simulink model "ClusterMG_1_SG"  (R2020a)
settings: Solver=FixedStepAuto  StartTime=0.0  StopTime=Tss  RelTol=1e-5  AbsTol=1e-5  EnableMultiTasking=on
values from neighbouring files (symbols this model uses):
  KA = K_sweep(cont)    [fault_tesis_1_SG.m]
  Ti = 1.5e-4    (= 0.00015)    [fault_tesis_1_SG.m]
  Tof = 1    [fault_tesis_1_SG.m]
undefined symbols (not defined in the file or in its folder): DiscIntNeverNeededParam, sigbuilder_block
libraries: powerlib x88, powerlib_meascontrol x49, simulink x20, spsExcitationSystemModel x1
(part 3 of 3)

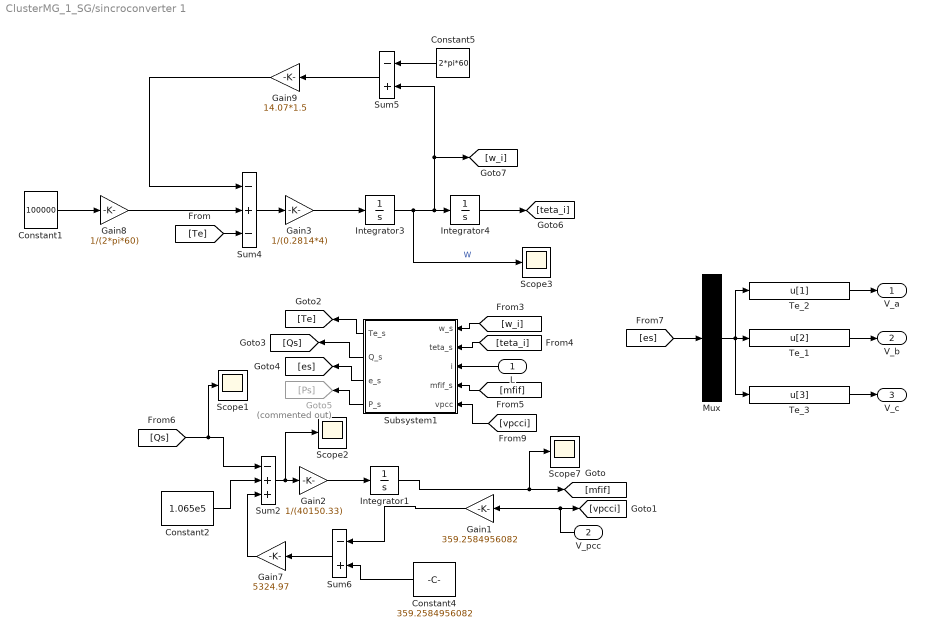
== system ClusterMG_1_SG/sincroconverter 1 ==
  L : Inport
  V_pcc : Inport  Port=2
  Constant1 : Constant  Value=100000
  Constant2 : Constant  Value=1.065e5
  Constant4 : Constant  Value=359.2584956082
  Constant5 : Constant  Value=2*pi*60
  Gain1 : Gain  Gain=359.2584956082
  Gain2 : Gain  Gain=1/(40150.33)
  Gain3 : Gain  Gain=1/(0.2814*4)
  Gain7 : Gain  Gain=5324.97
  Gain8 : Gain  Gain=1/(2*pi*60)
  Gain9 : Gain  Gain=14.07*1.5
  Goto5 : Goto  Commented=on  GotoTag=Ps
  Integrator1 : Integrator
  Integrator3 : Integrator  InitialCondition=376.9911
  Integrator4 : Integrator
  Mux : Mux  Inputs=1
  Scope{1..3,7} (4 alike) : Scope
  Subsystem1 : Subsystem
  Sum2 : Sum  Inputs=-++  InputSameDT=on  SaturateOnIntegerOverflow=on  OutDataTypeStr=Inherit: Same as first input
  Sum4 : Sum  Inputs=-+-  InputSameDT=on  SaturateOnIntegerOverflow=on  OutDataTypeStr=Inherit: Same as first input
  Sum5 : Sum  Inputs=-+  InputSameDT=on  SaturateOnIntegerOverflow=on  OutDataTypeStr=Inherit: Same as first input
  Sum6 : Sum  Inputs=-+  InputSameDT=on  SaturateOnIntegerOverflow=on  OutDataTypeStr=Inherit: Same as first input
  Te_1 : Fcn  Expr=u[2]
  Te_2 : Fcn  Expr=u[1]
  Te_3 : Fcn  Expr=u[3]
  V_a : Outport  VectorParamsAs1DForOutWhenUnconnected=off
  V_b : Outport  Port=2  VectorParamsAs1DForOutWhenUnconnected=off
  V_c : Outport  Port=3  VectorParamsAs1DForOutWhenUnconnected=off
  wires:
  Te_2/1 -> V_a/1
  Mux/1 -> Te_3/1, Te_2/1, Te_1/1
  Te_1/1 -> V_b/1
  Te_3/1 -> V_c/1
  [w_i] -> Subsystem1/1(w_s)
  [teta_i] -> Subsystem1/2(teta_s)
  [mfif] -> Subsystem1/4(mfif_s)
  Subsystem1/1(Te_s) -> [Te]
  Subsystem1/3(e_s) -> [es]
  Gain9/1 -> Sum4/1
  Sum4/1 -> Gain3/1
  Constant5/1 -> Sum5/1
  Integrator4/1 -> [teta_i]
  Sum5/1 -> Gain9/1
  Gain8/1 -> Sum4/2
  Gain3/1 -> Integrator3/1
  [Te] -> Sum4/3
  Gain7/1 -> Sum2/3
  Constant4/1 -> Sum6/2
  Gain2/1 -> Integrator1/1
  Sum6/1 -> Gain7/1
  Sum2/1 -> Scope2/1, Gain2/1
  L/1 -> Subsystem1/3(i)
  [es] -> Mux/1
  [Qs] -> Scope1/1, Sum2/1
  Subsystem1/4(P_s) -> Goto5/1
  Subsystem1/2(Q_s) -> [Qs]
  Constant2/1 -> Sum2/2
  Constant1/1 -> Gain8/1
  Integrator3/1 -> Scope3/1, Sum5/2, [w_i], Integrator4/1  "W"
  V_pcc/1 -> [vpcci], Gain1/1
  Integrator1/1 -> Scope7/1, [mfif]
  [vpcci] -> Subsystem1/5(vpcc)
  Gain1/1 -> Sum6/1

== system ClusterMG_1_SG/PLL/abc - qd ==
  a : Inport
  b : Inport  Port=2
  c : Inport  Port=3
  Gain : Gain  Gain=2/3
  Gain1 : Gain  Gain=-1/3
  Gain2 : Gain  Gain=-1/3
  Gain3 : Gain  Gain=1/sqrt(3)
  Gain4 : Gain  Gain=-1/sqrt(3)
  Sum : Sum  Inputs=|+++
  Sum1 : Sum  Inputs=|++
  d : Outport
  q : Outport  Port=2
  wires:
  Gain/1 -> Sum/1
  Gain1/1 -> Sum/2
  Gain2/1 -> Sum/3
  Gain4/1 -> Sum1/2
  Gain3/1 -> Sum1/1
  a/1 -> Gain/1
  b/1 -> Gain1/1, Gain3/1
  c/1 -> Gain2/1, Gain4/1
  Sum/1 -> d/1
  Sum1/1 -> q/1

== system ClusterMG_1_SG/PLL/qd - qe de1 ==
  vd : Inport
  vq : Inport  Port=2
  sin : Inport  Port=3
  cos : Inport  Port=4
  Gain : Gain  Gain=-1
  Product{1..4} (4 alike) : Product  RndMeth=Zero
  Sum1 : Sum  Inputs=|++
  Sum2 : Sum  Inputs=|++
  de : Outport
  qe : Outport  Port=2
  wires:
  Product2/1 -> Sum1/1
  Product3/1 -> Sum1/2
  vd/1 -> Product4/2, Product2/1
  vq/1 -> Product1/2, Product3/1
  Sum1/1 -> de/1
  cos/1 -> Product1/1, Product2/2
  sin/1 -> Gain/1, Product3/2
  Product4/1 -> Sum2/2
  Product1/1 -> Sum2/1
  Sum2/1 -> qe/1
  Gain/1 -> Product4/1

== system ClusterMG_1_SG/PLL2/abc - qd ==
  a : Inport
  b : Inport  Port=2
  c : Inport  Port=3
  Gain : Gain  Gain=2/3
  Gain1 : Gain  Gain=-1/3
  Gain2 : Gain  Gain=-1/3
  Gain3 : Gain  Gain=1/sqrt(3)
  Gain4 : Gain  Gain=-1/sqrt(3)
  Sum : Sum  Inputs=|+++
  Sum1 : Sum  Inputs=|++
  d : Outport
  q : Outport  Port=2
  wires:
  Gain/1 -> Sum/1
  Gain1/1 -> Sum/2
  Gain2/1 -> Sum/3
  Gain4/1 -> Sum1/2
  Gain3/1 -> Sum1/1
  a/1 -> Gain/1
  b/1 -> Gain1/1, Gain3/1
  c/1 -> Gain2/1, Gain4/1
  Sum/1 -> d/1
  Sum1/1 -> q/1

== system ClusterMG_1_SG/PLL2/qd - qe de1 ==
  vd : Inport
  vq : Inport  Port=2
  sin : Inport  Port=3
  cos : Inport  Port=4
  Gain : Gain  Gain=-1
  Product{1..4} (4 alike) : Product  RndMeth=Zero
  Sum1 : Sum  Inputs=|++
  Sum2 : Sum  Inputs=|++
  de : Outport
  qe : Outport  Port=2
  wires:
  Product2/1 -> Sum1/1
  Product3/1 -> Sum1/2
  vd/1 -> Product4/2, Product2/1
  vq/1 -> Product1/2, Product3/1
  Sum1/1 -> de/1
  cos/1 -> Product1/1, Product2/2
  sin/1 -> Gain/1, Product3/2
  Product4/1 -> Sum2/2
  Product1/1 -> Sum2/1
  Sum2/1 -> qe/1
  Gain/1 -> Product4/1

== system ClusterMG_1_SG/PLL3/abc - qd ==
  a : Inport
  b : Inport  Port=2
  c : Inport  Port=3
  Gain : Gain  Gain=2/3
  Gain1 : Gain  Gain=-1/3
  Gain2 : Gain  Gain=-1/3
  Gain3 : Gain  Gain=1/sqrt(3)
  Gain4 : Gain  Gain=-1/sqrt(3)
  Sum : Sum  Inputs=|+++
  Sum1 : Sum  Inputs=|++
  d : Outport
  q : Outport  Port=2
  wires:
  Gain/1 -> Sum/1
  Gain1/1 -> Sum/2
  Gain2/1 -> Sum/3
  Gain4/1 -> Sum1/2
  Gain3/1 -> Sum1/1
  a/1 -> Gain/1
  b/1 -> Gain1/1, Gain3/1
  c/1 -> Gain2/1, Gain4/1
  Sum/1 -> d/1
  Sum1/1 -> q/1

== system ClusterMG_1_SG/PLL3/qd - qe de1 ==
  vd : Inport
  vq : Inport  Port=2
  sin : Inport  Port=3
  cos : Inport  Port=4
  Gain : Gain  Gain=-1
  Product{1..4} (4 alike) : Product  RndMeth=Zero
  Sum1 : Sum  Inputs=|++
  Sum2 : Sum  Inputs=|++
  de : Outport
  qe : Outport  Port=2
  wires:
  Product2/1 -> Sum1/1
  Product3/1 -> Sum1/2
  vd/1 -> Product4/2, Product2/1
  vq/1 -> Product1/2, Product3/1
  Sum1/1 -> de/1
  cos/1 -> Product1/1, Product2/2
  sin/1 -> Gain/1, Product3/2
  Product4/1 -> Sum2/2
  Product1/1 -> Sum2/1
  Sum2/1 -> qe/1
  Gain/1 -> Product4/1

== system ClusterMG_1_SG/PLL4/abc - qd ==
  a : Inport
  b : Inport  Port=2
  c : Inport  Port=3
  Gain : Gain  Gain=2/3
  Gain1 : Gain  Gain=-1/3
  Gain2 : Gain  Gain=-1/3
  Gain3 : Gain  Gain=1/sqrt(3)
  Gain4 : Gain  Gain=-1/sqrt(3)
  Sum : Sum  Inputs=|+++
  Sum1 : Sum  Inputs=|++
  d : Outport
  q : Outport  Port=2
  wires:
  Gain/1 -> Sum/1
  Gain1/1 -> Sum/2
  Gain2/1 -> Sum/3
  Gain4/1 -> Sum1/2
  Gain3/1 -> Sum1/1
  a/1 -> Gain/1
  b/1 -> Gain1/1, Gain3/1
  c/1 -> Gain2/1, Gain4/1
  Sum/1 -> d/1
  Sum1/1 -> q/1

== system ClusterMG_1_SG/PLL4/qd - qe de1 ==
  vd : Inport
  vq : Inport  Port=2
  sin : Inport  Port=3
  cos : Inport  Port=4
  Gain : Gain  Gain=-1
  Product{1..4} (4 alike) : Product  RndMeth=Zero
  Sum1 : Sum  Inputs=|++
  Sum2 : Sum  Inputs=|++
  de : Outport
  qe : Outport  Port=2
  wires:
  Product2/1 -> Sum1/1
  Product3/1 -> Sum1/2
  vd/1 -> Product4/2, Product2/1
  vq/1 -> Product1/2, Product3/1
  Sum1/1 -> de/1
  cos/1 -> Product1/1, Product2/2
  sin/1 -> Gain/1, Product3/2
  Product4/1 -> Sum2/2
  Product1/1 -> Sum2/1
  Sum2/1 -> qe/1
  Gain/1 -> Product4/1

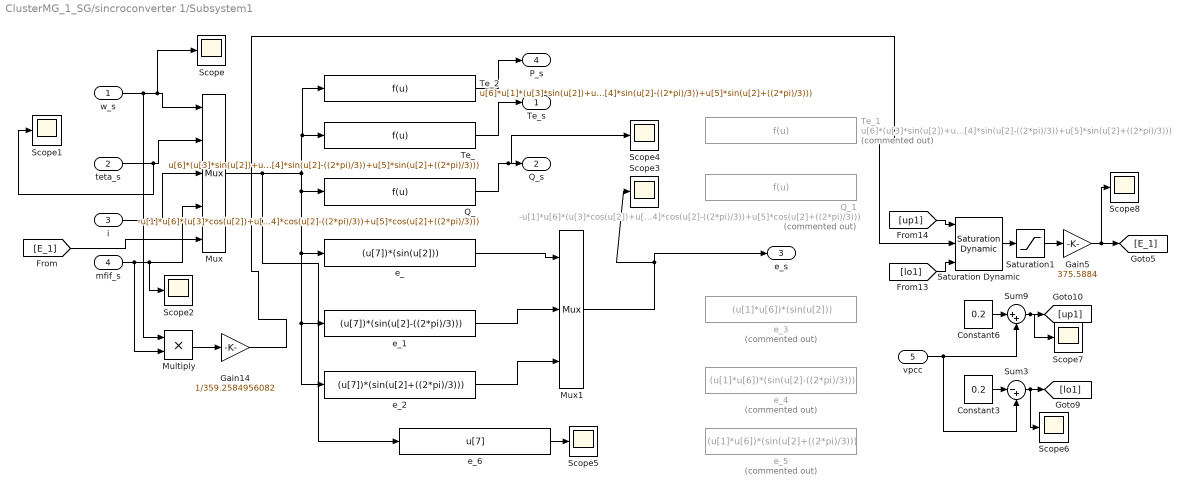
== system ClusterMG_1_SG/sincroconverter 1/Subsystem1 ==
  w_s : Inport
  teta_s : Inport  Port=2
  i : Inport  Port=3
  mfif_s : Inport  Port=4
  vpcc : Inport  Port=5
  Constant3 : Constant  Value=0.2
  Constant6 : Constant  Value=0.2
  Gain14 : Gain  Gain=1/359.2584956082
  Gain5 : Gain  Gain=375.5884
  Multiply : Product
  Mux : Mux  Inputs=5
  Mux1 : Mux  Inputs=3
  Q_ : Fcn  Expr=-u[1]*u[6]*(u[3]*cos(u[2])+u[4]*cos(u[2]-((2*pi)/3))+u[5]*cos(u[2]+((2*pi)/3)))
  Q_1 : Fcn  Commented=on  Expr=-u[1]*u[6]*(u[3]*cos(u[2])+u[4]*cos(u[2]-((2*pi)/3))+u[5]*cos(u[2]+((2*pi)/3)))
  Saturation Dynamic : simulink/Discontinuities/Saturation Dynamic  OutMin=[]  OutMax=[]  OutDataTypeStr=Inherit: Same as second input  OutDataType=fixdt(1, 16)  OutScaling=2^-10  DoSatur=off
  Saturation1 : Saturate  UpperLimit=1.21  LowerLimit=0
  Scope{,1..8} (9 alike) : Scope
  Sum3 : Sum  Inputs=|-+
  Sum9 : Sum  Inputs=|++
  Te_ : Fcn  Expr=u[6]*(u[3]*sin(u[2])+u[4]*sin(u[2]-((2*pi)/3))+u[5]*sin(u[2]+((2*pi)/3)))
  Te_1 : Fcn  Commented=on  Expr=u[6]*(u[3]*sin(u[2])+u[4]*sin(u[2]-((2*pi)/3))+u[5]*sin(u[2]+((2*pi)/3)))
  Te_2 : Fcn  Expr=u[6]*u[1]*(u[3]*sin(u[2])+u[4]*sin(u[2]-((2*pi)/3))+u[5]*sin(u[2]+((2*pi)/3)))
  e_ : Fcn  Expr=(u[7])*(sin(u[2]))
  e_1 : Fcn  Expr=(u[7])*(sin(u[2]-((2*pi)/3)))
  e_2 : Fcn  Expr=(u[7])*(sin(u[2]+((2*pi)/3)))
  e_3 : Fcn  Commented=on  Expr=(u[1]*u[6])*(sin(u[2]))
  e_4 : Fcn  Commented=on  Expr=(u[1]*u[6])*(sin(u[2]-((2*pi)/3)))
  e_5 : Fcn  Commented=on  Expr=(u[1]*u[6])*(sin(u[2]+((2*pi)/3)))
  e_6 : Fcn  Expr=u[7]
  Te_s : Outport  VectorParamsAs1DForOutWhenUnconnected=off
  Q_s : Outport  Port=2  VectorParamsAs1DForOutWhenUnconnected=off
  e_s : Outport  Port=3  VectorParamsAs1DForOutWhenUnconnected=off
  P_s : Outport  Port=4  VectorParamsAs1DForOutWhenUnconnected=off
  wires:
  i/1 -> Mux/3
  Mux/1 -> e_6/1, e_2/1, e_1/1, e_/1, Q_/1, Te_2/1, Te_/1
  Te_/1 -> Te_s/1
  Q_/1 -> Scope4/1, Q_s/1
  teta_s/1 -> Scope1/1, Mux/2
  Te_2/1 -> P_s/1
  e_/1 -> Mux1/1
  e_1/1 -> Mux1/2
  e_2/1 -> Mux1/3
  Mux1/1 -> Scope3/1, e_s/1
  w_s/1 -> Multiply/1, Scope/1, Mux/1
  mfif_s/1 -> Multiply/2, Scope2/1, Mux/4
  Multiply/1 -> Gain14/1
  e_6/1 -> Scope5/1
  [up1] -> Saturation Dynamic/1
  [lo1] -> Saturation Dynamic/3
  Gain5/1 -> Scope8/1, [E_1]
  Gain14/1 -> Saturation Dynamic/2
  Constant6/1 -> Sum9/1
  Constant3/1 -> Sum3/1
  Sum9/1 -> Scope7/1, [up1]
  vpcc/1 -> Sum3/2, Sum9/2
  Sum3/1 -> [lo1], Scope6/1
  [E_1] -> Mux/5
  Saturation Dynamic/1 -> Saturation1/1
  Saturation1/1 -> Gain5/1
